simulink model "p5p5ex"  (Simulink 9.1)
settings: Solver=VariableStepAuto  StartTime=0.0  StopTime=500  FixedStep=timestep  RelTol=1e-3  EnableMultiTasking=on
values from neighbouring files (symbols this model uses):
  psi_r = 30    [p5p5d.m]
  T_s = 0.1    [p5p5a.m]
undefined symbols (not defined in the file or in its folder): K_pd, T_d, T_f
libraries: simulink x2
settings Model: SuppressorTable=22 serialization::archive 11 0 6 0 0 0 0 0  Creator=markh  LastModifiedBy=bernhardpg
settings DataIOCC: LimitDataPoints=on  SignalLoggingSaveFormat=ModelDataLogs  SignalLoggingName=sigsOut
settings OptimizationCC: InitFltsAndDblsToZero=on
settings DebuggingCC: SaveWithParameterizedLinksMsg=none  SignalResolutionControl=TryResolveAllWithWarning  MultiTaskDSMMsg=warning  MultiTaskCondExecSysMsg=none  FcnCallInpInsideContextMsg=warning  StateNameClashWarn=warning
settings HardwareCC: TargetUnknown=on
settings GRTTargetCC: TargetFcnLib=ansi_tfl_tmw.mat  GeneratePreprocessorConditionals=Disable all

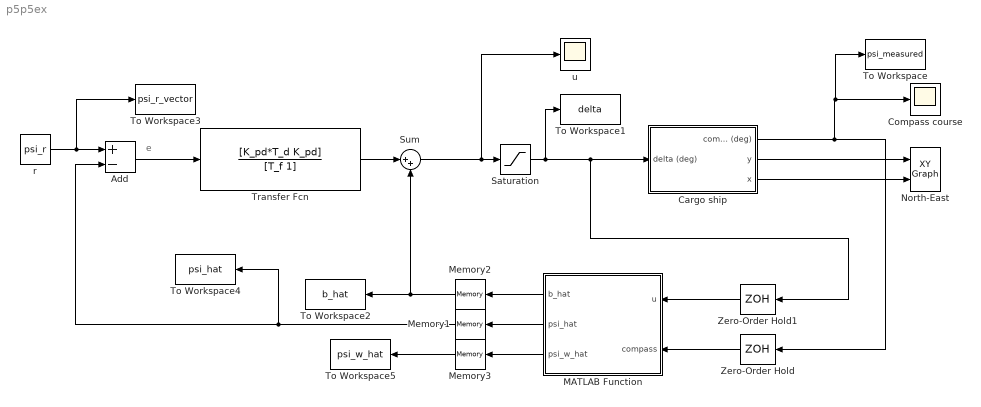
== system p5p5ex ==
  note: e
  Add : Sum  Inputs=+-
  Cargo ship : Subsystem  mask(Simple shipmodel for a cargo ship){noise=on, current=on, logic=on}
      mask prompts: noise "measurement noise"; logic "waves"
      mask help:
      | Measurement noise:
      | 	checked = noise on
      | 	unchecked = noise off
      |
      | Current:
      | 	checked = current on
      | 	unchecked = current off
      |
      | Waves:
      | 	checked = waves on
      | 	unchecked = waves off
      |
      | Author: Jørgen Spjøtvold, 9/10-2003
      | TTK 4115 Linear system theory.
      | Modified by Jostein Bakkeheim 26/10-2006
  Compass course : Scope
  MATLAB Function : MATLAB Function  TreatAsAtomicUnit=on
  Memory1 : Memory
  Memory2 : Memory
  Memory3 : Memory
  North-East : simulink/Sinks/XY Graph  xmin=-5000  xmax=5000  ymin=-5000  ymax=5000  st=-1
  Saturation : Saturate  UpperLimit=35  LowerLimit=-35
  Sum : Sum  Inputs=|++
  To Workspace : ToWorkspace  VariableName=psi_measured  SaveFormat=Timeseries  SampleTime=-1
  To Workspace1 : ToWorkspace  VariableName=delta  SaveFormat=Timeseries  SampleTime=-1
  To Workspace2 : ToWorkspace  VariableName=b_hat  SaveFormat=Timeseries  SampleTime=-1
  To Workspace3 : ToWorkspace  VariableName=psi_r_vector  SaveFormat=Timeseries  SampleTime=-1
  To Workspace4 : ToWorkspace  VariableName=psi_hat  SaveFormat=Timeseries  SampleTime=-1
  To Workspace5 : ToWorkspace  VariableName=psi_w_hat  SaveFormat=Timeseries  SampleTime=-1
  Transfer Fcn : TransferFcn  Numerator=[K_pd*T_d K_pd]  Denominator=[T_f 1]
  Zero-Order Hold : ZeroOrderHold  SampleTime=T_s
  Zero-Order Hold1 : ZeroOrderHold  SampleTime=T_s
  r : Constant  Value=psi_r
  u : Scope
  wires:
  Cargo ship/3(x) -> North-East/2
  Cargo ship/2(y) -> North-East/1
  r/1 -> To Workspace3/1, Add/1
  Add/1 -> Transfer Fcn/1
  Zero-Order Hold/1 -> MATLAB Function/2(compass)
  Zero-Order Hold1/1 -> MATLAB Function/1(u)
  Transfer Fcn/1 -> Sum/1
  MATLAB Function/1(b_hat) -> Memory2/1
  Sum/1 -> u/1, Saturation/1
  Saturation/1 -> Zero-Order Hold1/1, Cargo ship/1(delta (deg)), To Workspace1/1
  Memory2/1 -> To Workspace2/1, Sum/2
  MATLAB Function/2(psi_hat) -> Memory1/1
  Memory1/1 -> To Workspace4/1, Add/2
  MATLAB Function/3(psi_w_hat) -> Memory3/1
  Memory3/1 -> To Workspace5/1
  Cargo ship/1(compass (deg)) -> Zero-Order Hold/1, To Workspace/1, Compass course/1

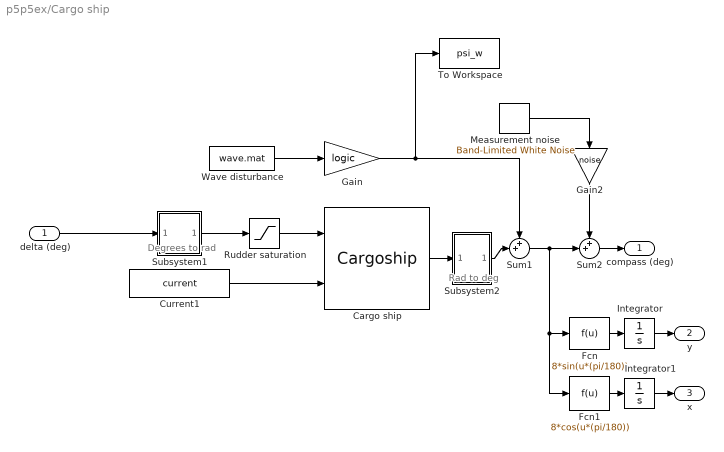
== system p5p5ex/Cargo ship ==
  note: Degrees to rad
  note: Rad to deg
  delta (deg) : Inport
  Cargo ship : S-Function  FunctionName=Cargoship  SFunctionDeploymentMode=off  EnableBusSupport=off  mask(Cargo ship){}
      mask help:
      | S-function which simulates a cargo ship.
      |
      | Author: Jørgen Spjøtvold
      | 20.10-2003
      | Modified by Jostein Bakkeheim 27.10.2006
  Current1 : Constant  Value=current
  Fcn : Fcn  Expr=8*sin(u*(pi/180))
  Fcn1 : Fcn  Expr=8*cos(u*(pi/180))
  Gain : Gain  Gain=logic  SaturateOnIntegerOverflow=on  OutDataTypeStr=Inherit: Same as input  ParamDataTypeStr=Inherit: Same as input
  Gain2 : Gain  Gain=noise  SaturateOnIntegerOverflow=on  OutDataTypeStr=Inherit: Same as input  ParamDataTypeStr=Inherit: Same as input
  Integrator : Integrator
  Integrator1 : Integrator
  Measurement noise : simulink/Sources/Band-Limited White Noise  Cov=[0.001]  Ts=.5  seed=[23341]
  Rudder saturation : Saturate  UpperLimit=45*(pi/180)  LowerLimit=-45*(pi/180)
  Subsystem1 : Subsystem  mask(degrees to radians){}
      mask help: Converts degrees to radians
      mask Display: fprintf('D2R');
  Subsystem2 : Subsystem  mask(radians to degrees){}
      mask help: Converts radians to degrees
      mask Display: fprintf('R2D');
  Sum1 : Sum  Inputs=++|  SaturateOnIntegerOverflow=on
  Sum2 : Sum  Inputs=++|  SaturateOnIntegerOverflow=on
  To Workspace : ToWorkspace  VariableName=psi_w  SaveFormat=Timeseries  SampleTime=-1
  Wave disturbance : FromFile  FileName=wave.mat  SampleTime=0
  compass (deg) : Outport
  y : Outport  Port=2
  x : Outport  Port=3
  wires:
  delta (deg)/1 -> Subsystem1/1(In1)
  Fcn/1 -> Integrator/1
  Integrator/1 -> y/1
  Fcn1/1 -> Integrator1/1
  Integrator1/1 -> x/1
  Wave disturbance/1 -> Gain/1
  Subsystem2/1(Out1) -> Sum1/2
  Gain/1 -> To Workspace/1, Sum1/1
  Sum1/1 -> Fcn/1, Fcn1/1, Sum2/2
  Cargo ship/1 -> Subsystem2/1(In1)
  Subsystem1/1(Out1) -> Rudder saturation/1
  Rudder saturation/1 -> Cargo ship/1
  Sum2/1 -> compass (deg)/1
  Measurement noise/1 -> Gain2/1
  Gain2/1 -> Sum2/1
  Current1/1 -> Cargo ship/2

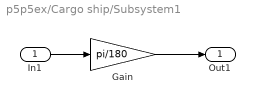
== system p5p5ex/Cargo ship/Subsystem1 ==
  In1 : Inport
  Gain : Gain  Gain=pi/180  SaturateOnIntegerOverflow=on  OutDataTypeStr=Inherit: Same as input  ParamDataTypeStr=Inherit: Same as input
  Out1 : Outport
  wires:
  Gain/1 -> Out1/1
  In1/1 -> Gain/1

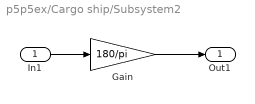
== system p5p5ex/Cargo ship/Subsystem2 ==
  In1 : Inport
  Gain : Gain  Gain=180/pi  SaturateOnIntegerOverflow=on  OutDataTypeStr=Inherit: Same as input  ParamDataTypeStr=Inherit: Same as input
  Out1 : Outport
  wires:
  Gain/1 -> Out1/1
  In1/1 -> Gain/1

== matlab function MATLAB Function ==
  data: b_hat output double; u input double; compass input double; psi_hat output double; system parameter double; psi_w_hat output double
function [b_hat, psi_hat, psi_w_hat]   = fcn(u, compass, system)

persistent init_flag A_d B_d C_d E_d R Q x_hat_k_apriori P_k_apriori

if isempty(init_flag)
    init_flag = 1;
    [A_d, B_d, C_d, E_d, R, Q, x_hat_k_apriori, P_k_apriori] = ...
        deal(system.A_d, system.B_d, system.C_d, system.E_d, ...
        system.R, system.Q, ...
        system.x_hat_0_apriori, system.P_0_apriori);
end

% Compute Kalman gain
K_k = P_k_apriori * C_d' * inv(C_d * P_k_apriori * C_d' + R);

% Update estimate with measurement
x_hat_k = x_hat_k_apriori + K_k * (compass - C_d * x_hat_k_apriori);

% Compute error covariance for updated estimate
%P_k = (eye(5) - K_k * C_d) * P_k_apriori;
P_k = (eye(5) - K_k * C_d) * P_k_apriori * (eye(5) - K_k * C_d)' + K_k * R * K_k';

% Project ahead
x_hat_k_apriori = A_d * x_hat_k + B_d * u;
P_k_apriori = A_d * P_k * A_d' + E_d * Q * E_d';

psi_hat = x_hat_k(3);
b_hat = x_hat_k(5);
psi_w_hat = x_hat_k(2);
